simulink model "Subtractor4bit"  (R2025b)
settings: Solver=VariableStepAuto  StartTime=0.0  StopTime=10.0  RelTol=1e-3
settings Model: Creator=cyber  LastModifiedBy=cyber

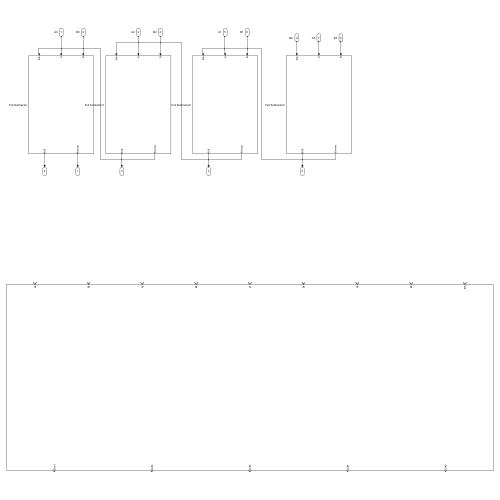
[thumbnail: Simulink's stored preview of the top-level diagram]
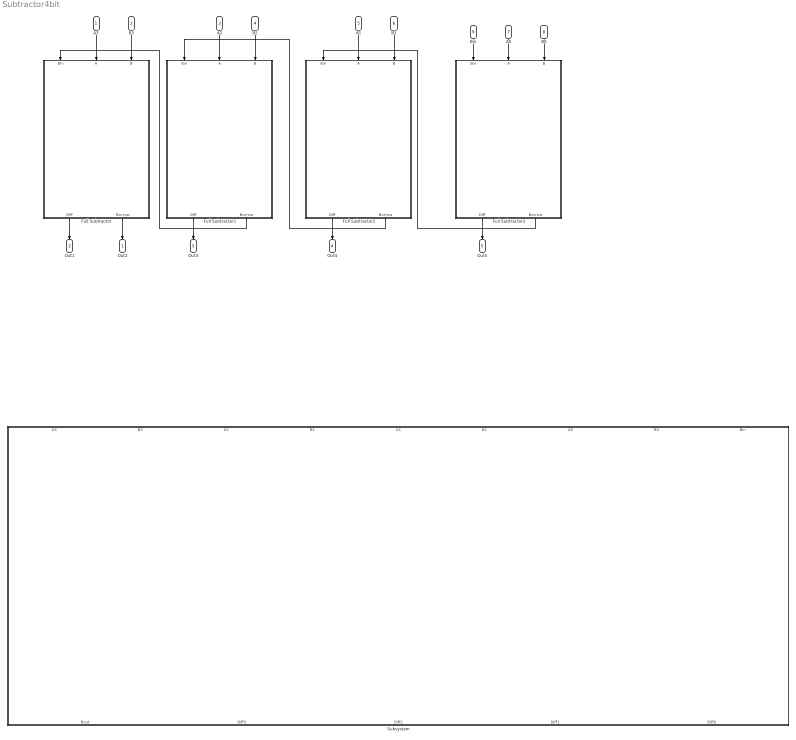
== system Subtractor4bit ==
  A3 : Inport
  B3 : Inport  Port=2
  A2 : Inport  Port=3
  B2 : Inport  Port=4
  A1 : Inport  Port=5
  B1 : Inport  Port=6
  A0 : Inport  Port=7
  B0 : Inport  Port=8
  Bin : Inport  Port=9
  Full Subtractor : Subsystem
  Full Subtractor1 : Subsystem
  Full Subtractor2 : Subsystem
  Full Subtractor3 : Subsystem
  Subsystem : Subsystem
  Out2 : Outport
  Out1 : Outport  Port=2
  Out3 : Outport  Port=3
  Out4 : Outport  Port=4
  Out5 : Outport  Port=5
  wires:
  Full Subtractor/1(Diff) -> Out1/1
  Full Subtractor1/1(Diff) -> Out3/1
  Full Subtractor2/1(Diff) -> Out4/1
  Full Subtractor3/1(Diff) -> Out5/1
  Full Subtractor3/2(Borrow) -> Full Subtractor2/1(Bin)
  Full Subtractor2/2(Borrow) -> Full Subtractor1/1(Bin)
  Full Subtractor1/2(Borrow) -> Full Subtractor/1(Bin)
  A3/1 -> Full Subtractor/2(A)
  B3/1 -> Full Subtractor/3(B)
  A2/1 -> Full Subtractor1/2(A)
  B2/1 -> Full Subtractor1/3(B)
  A1/1 -> Full Subtractor2/2(A)
  B1/1 -> Full Subtractor2/3(B)
  Full Subtractor/2(Borrow) -> Out2/1
  A0/1 -> Full Subtractor3/2(A)
  B0/1 -> Full Subtractor3/3(B)
  Bin/1 -> Full Subtractor3/1(Bin)

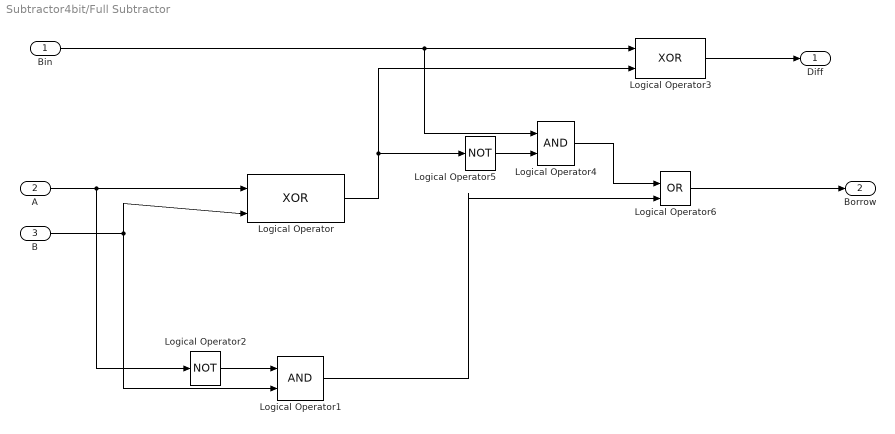
== system Subtractor4bit/Full Subtractor ==
  Bin : Inport
  A : Inport  Port=2
  B : Inport  Port=3
  Logical Operator : Logic  Operator=XOR  IconShape=distinctive  AllPortsSameDT=off  OutDataTypeStr=boolean
  Logical Operator1 : Logic  IconShape=distinctive  AllPortsSameDT=off  OutDataTypeStr=boolean
  Logical Operator2 : Logic  Operator=NOT  IconShape=distinctive  AllPortsSameDT=off  OutDataTypeStr=boolean
  Logical Operator3 : Logic  Operator=XOR  IconShape=distinctive  AllPortsSameDT=off  OutDataTypeStr=boolean
  Logical Operator4 : Logic  IconShape=distinctive  AllPortsSameDT=off  OutDataTypeStr=boolean
  Logical Operator5 : Logic  Operator=NOT  IconShape=distinctive  AllPortsSameDT=off  OutDataTypeStr=boolean
  Logical Operator6 : Logic  Operator=OR  IconShape=distinctive  AllPortsSameDT=off  OutDataTypeStr=boolean
  Diff : Outport
  Borrow : Outport  Port=2
  wires:
  Logical Operator/1 -> Logical Operator3/2, Logical Operator5/1
  Logical Operator1/1 -> Logical Operator6/2
  A/1 -> Logical Operator2/1, Logical Operator/1
  Bin/1 -> Logical Operator4/1, Logical Operator3/1
  Logical Operator3/1 -> Diff/1
  B/1 -> Logical Operator/2, Logical Operator1/2
  Logical Operator2/1 -> Logical Operator1/1
  Logical Operator4/1 -> Logical Operator6/1
  Logical Operator5/1 -> Logical Operator4/2
  Logical Operator6/1 -> Borrow/1

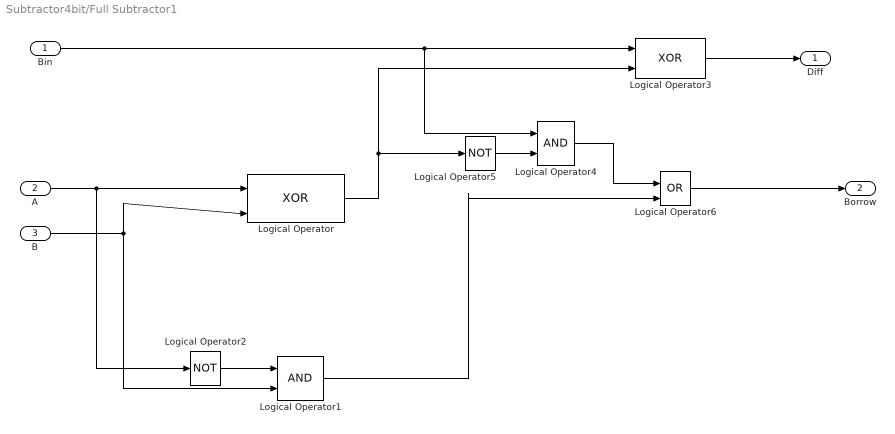
== system Subtractor4bit/Full Subtractor1 ==
  Bin : Inport
  A : Inport  Port=2
  B : Inport  Port=3
  Logical Operator : Logic  Operator=XOR  IconShape=distinctive  AllPortsSameDT=off  OutDataTypeStr=boolean
  Logical Operator1 : Logic  IconShape=distinctive  AllPortsSameDT=off  OutDataTypeStr=boolean
  Logical Operator2 : Logic  Operator=NOT  IconShape=distinctive  AllPortsSameDT=off  OutDataTypeStr=boolean
  Logical Operator3 : Logic  Operator=XOR  IconShape=distinctive  AllPortsSameDT=off  OutDataTypeStr=boolean
  Logical Operator4 : Logic  IconShape=distinctive  AllPortsSameDT=off  OutDataTypeStr=boolean
  Logical Operator5 : Logic  Operator=NOT  IconShape=distinctive  AllPortsSameDT=off  OutDataTypeStr=boolean
  Logical Operator6 : Logic  Operator=OR  IconShape=distinctive  AllPortsSameDT=off  OutDataTypeStr=boolean
  Diff : Outport
  Borrow : Outport  Port=2
  wires:
  Logical Operator/1 -> Logical Operator3/2, Logical Operator5/1
  Logical Operator1/1 -> Logical Operator6/2
  A/1 -> Logical Operator2/1, Logical Operator/1
  Bin/1 -> Logical Operator4/1, Logical Operator3/1
  Logical Operator3/1 -> Diff/1
  B/1 -> Logical Operator/2, Logical Operator1/2
  Logical Operator2/1 -> Logical Operator1/1
  Logical Operator4/1 -> Logical Operator6/1
  Logical Operator5/1 -> Logical Operator4/2
  Logical Operator6/1 -> Borrow/1

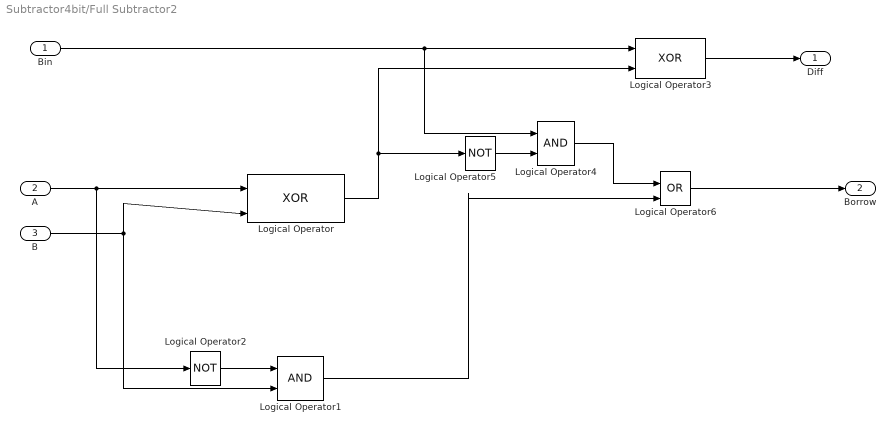
== system Subtractor4bit/Full Subtractor2 ==
  Bin : Inport
  A : Inport  Port=2
  B : Inport  Port=3
  Logical Operator : Logic  Operator=XOR  IconShape=distinctive  AllPortsSameDT=off  OutDataTypeStr=boolean
  Logical Operator1 : Logic  IconShape=distinctive  AllPortsSameDT=off  OutDataTypeStr=boolean
  Logical Operator2 : Logic  Operator=NOT  IconShape=distinctive  AllPortsSameDT=off  OutDataTypeStr=boolean
  Logical Operator3 : Logic  Operator=XOR  IconShape=distinctive  AllPortsSameDT=off  OutDataTypeStr=boolean
  Logical Operator4 : Logic  IconShape=distinctive  AllPortsSameDT=off  OutDataTypeStr=boolean
  Logical Operator5 : Logic  Operator=NOT  IconShape=distinctive  AllPortsSameDT=off  OutDataTypeStr=boolean
  Logical Operator6 : Logic  Operator=OR  IconShape=distinctive  AllPortsSameDT=off  OutDataTypeStr=boolean
  Diff : Outport
  Borrow : Outport  Port=2
  wires:
  Logical Operator/1 -> Logical Operator3/2, Logical Operator5/1
  Logical Operator1/1 -> Logical Operator6/2
  A/1 -> Logical Operator2/1, Logical Operator/1
  Bin/1 -> Logical Operator4/1, Logical Operator3/1
  Logical Operator3/1 -> Diff/1
  B/1 -> Logical Operator/2, Logical Operator1/2
  Logical Operator2/1 -> Logical Operator1/1
  Logical Operator4/1 -> Logical Operator6/1
  Logical Operator5/1 -> Logical Operator4/2
  Logical Operator6/1 -> Borrow/1

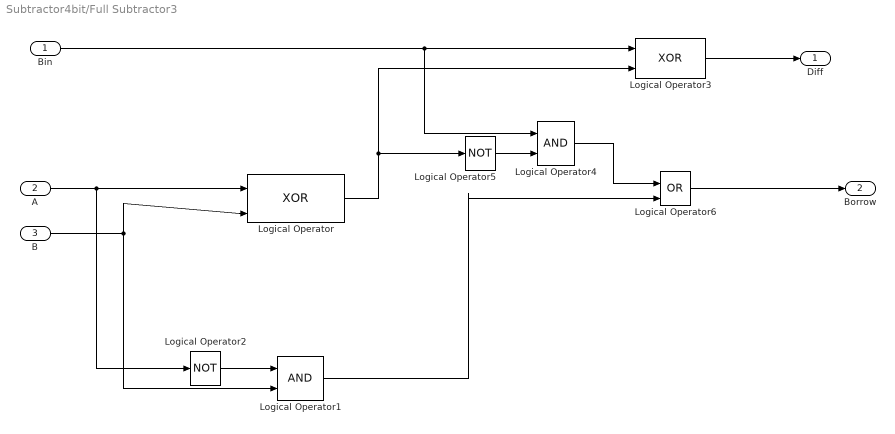
== system Subtractor4bit/Full Subtractor3 ==
  Bin : Inport
  A : Inport  Port=2
  B : Inport  Port=3
  Logical Operator : Logic  Operator=XOR  IconShape=distinctive  AllPortsSameDT=off  OutDataTypeStr=boolean
  Logical Operator1 : Logic  IconShape=distinctive  AllPortsSameDT=off  OutDataTypeStr=boolean
  Logical Operator2 : Logic  Operator=NOT  IconShape=distinctive  AllPortsSameDT=off  OutDataTypeStr=boolean
  Logical Operator3 : Logic  Operator=XOR  IconShape=distinctive  AllPortsSameDT=off  OutDataTypeStr=boolean
  Logical Operator4 : Logic  IconShape=distinctive  AllPortsSameDT=off  OutDataTypeStr=boolean
  Logical Operator5 : Logic  Operator=NOT  IconShape=distinctive  AllPortsSameDT=off  OutDataTypeStr=boolean
  Logical Operator6 : Logic  Operator=OR  IconShape=distinctive  AllPortsSameDT=off  OutDataTypeStr=boolean
  Diff : Outport
  Borrow : Outport  Port=2
  wires:
  Logical Operator/1 -> Logical Operator3/2, Logical Operator5/1
  Logical Operator1/1 -> Logical Operator6/2
  A/1 -> Logical Operator2/1, Logical Operator/1
  Bin/1 -> Logical Operator4/1, Logical Operator3/1
  Logical Operator3/1 -> Diff/1
  B/1 -> Logical Operator/2, Logical Operator1/2
  Logical Operator2/1 -> Logical Operator1/1
  Logical Operator4/1 -> Logical Operator6/1
  Logical Operator5/1 -> Logical Operator4/2
  Logical Operator6/1 -> Borrow/1

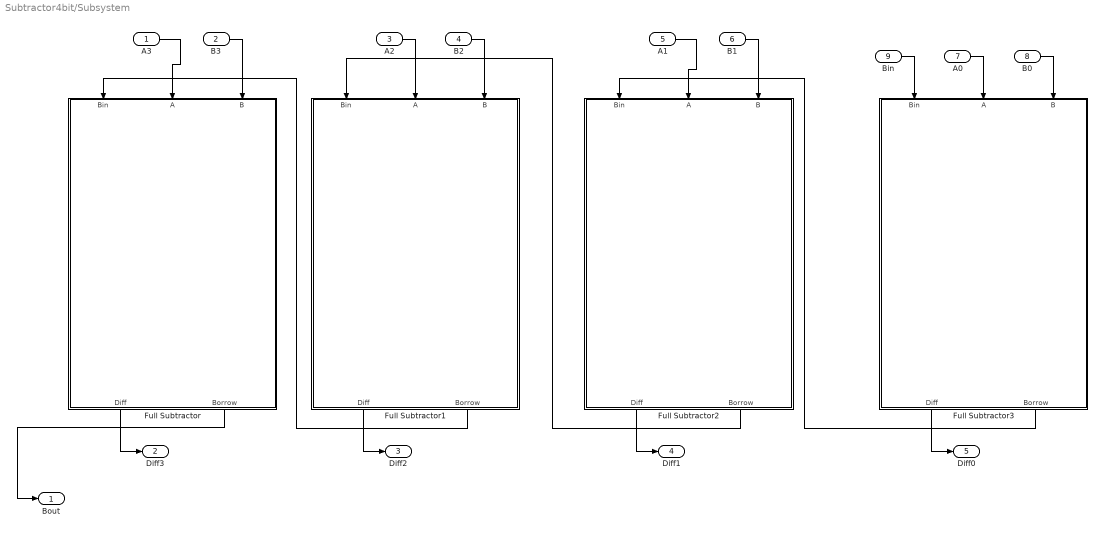
== system Subtractor4bit/Subsystem ==
  A3 : Inport
  B3 : Inport  Port=2
  A2 : Inport  Port=3
  B2 : Inport  Port=4
  A1 : Inport  Port=5
  B1 : Inport  Port=6
  A0 : Inport  Port=7
  B0 : Inport  Port=8
  Bin : Inport  Port=9
  Full Subtractor : Subsystem
  Full Subtractor1 : Subsystem
  Full Subtractor2 : Subsystem
  Full Subtractor3 : Subsystem
  Bout : Outport
  Diff3 : Outport  Port=2
  Diff2 : Outport  Port=3
  Diff1 : Outport  Port=4
  Diff0 : Outport  Port=5
  wires:
  Full Subtractor1/1(Diff) -> Diff2/1
  Full Subtractor2/1(Diff) -> Diff1/1
  Full Subtractor3/2(Borrow) -> Full Subtractor2/1(Bin)
  Full Subtractor2/2(Borrow) -> Full Subtractor1/1(Bin)
  Full Subtractor1/2(Borrow) -> Full Subtractor/1(Bin)
  B3/1 -> Full Subtractor/3(B)
  A0/1 -> Full Subtractor3/2(A)
  A2/1 -> Full Subtractor1/2(A)
  Full Subtractor/2(Borrow) -> Bout/1
  Full Subtractor3/1(Diff) -> Diff0/1
  A3/1 -> Full Subtractor/2(A)
  B2/1 -> Full Subtractor1/3(B)
  A1/1 -> Full Subtractor2/2(A)
  B1/1 -> Full Subtractor2/3(B)
  Bin/1 -> Full Subtractor3/1(Bin)
  Full Subtractor/1(Diff) -> Diff3/1
  B0/1 -> Full Subtractor3/3(B)

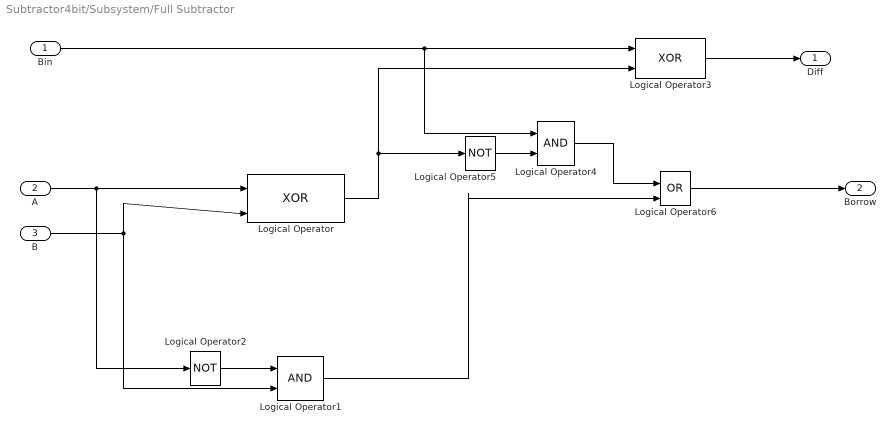
== system Subtractor4bit/Subsystem/Full Subtractor ==
  Bin : Inport
  A : Inport  Port=2
  B : Inport  Port=3
  Logical Operator : Logic  Operator=XOR  IconShape=distinctive  AllPortsSameDT=off  OutDataTypeStr=boolean
  Logical Operator1 : Logic  IconShape=distinctive  AllPortsSameDT=off  OutDataTypeStr=boolean
  Logical Operator2 : Logic  Operator=NOT  IconShape=distinctive  AllPortsSameDT=off  OutDataTypeStr=boolean
  Logical Operator3 : Logic  Operator=XOR  IconShape=distinctive  AllPortsSameDT=off  OutDataTypeStr=boolean
  Logical Operator4 : Logic  IconShape=distinctive  AllPortsSameDT=off  OutDataTypeStr=boolean
  Logical Operator5 : Logic  Operator=NOT  IconShape=distinctive  AllPortsSameDT=off  OutDataTypeStr=boolean
  Logical Operator6 : Logic  Operator=OR  IconShape=distinctive  AllPortsSameDT=off  OutDataTypeStr=boolean
  Diff : Outport
  Borrow : Outport  Port=2
  wires:
  Logical Operator/1 -> Logical Operator3/2, Logical Operator5/1
  Logical Operator1/1 -> Logical Operator6/2
  A/1 -> Logical Operator2/1, Logical Operator/1
  Bin/1 -> Logical Operator4/1, Logical Operator3/1
  Logical Operator3/1 -> Diff/1
  B/1 -> Logical Operator/2, Logical Operator1/2
  Logical Operator2/1 -> Logical Operator1/1
  Logical Operator4/1 -> Logical Operator6/1
  Logical Operator5/1 -> Logical Operator4/2
  Logical Operator6/1 -> Borrow/1

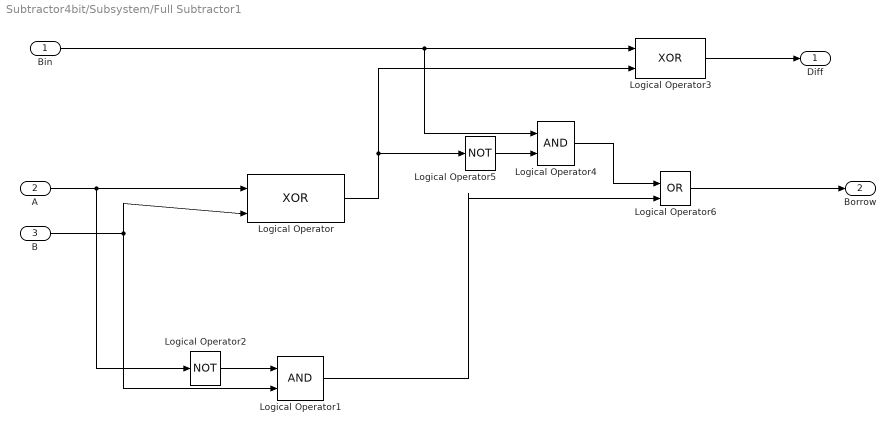
== system Subtractor4bit/Subsystem/Full Subtractor1 ==
  Bin : Inport
  A : Inport  Port=2
  B : Inport  Port=3
  Logical Operator : Logic  Operator=XOR  IconShape=distinctive  AllPortsSameDT=off  OutDataTypeStr=boolean
  Logical Operator1 : Logic  IconShape=distinctive  AllPortsSameDT=off  OutDataTypeStr=boolean
  Logical Operator2 : Logic  Operator=NOT  IconShape=distinctive  AllPortsSameDT=off  OutDataTypeStr=boolean
  Logical Operator3 : Logic  Operator=XOR  IconShape=distinctive  AllPortsSameDT=off  OutDataTypeStr=boolean
  Logical Operator4 : Logic  IconShape=distinctive  AllPortsSameDT=off  OutDataTypeStr=boolean
  Logical Operator5 : Logic  Operator=NOT  IconShape=distinctive  AllPortsSameDT=off  OutDataTypeStr=boolean
  Logical Operator6 : Logic  Operator=OR  IconShape=distinctive  AllPortsSameDT=off  OutDataTypeStr=boolean
  Diff : Outport
  Borrow : Outport  Port=2
  wires:
  Logical Operator/1 -> Logical Operator3/2, Logical Operator5/1
  Logical Operator1/1 -> Logical Operator6/2
  A/1 -> Logical Operator2/1, Logical Operator/1
  Bin/1 -> Logical Operator4/1, Logical Operator3/1
  Logical Operator3/1 -> Diff/1
  B/1 -> Logical Operator/2, Logical Operator1/2
  Logical Operator2/1 -> Logical Operator1/1
  Logical Operator4/1 -> Logical Operator6/1
  Logical Operator5/1 -> Logical Operator4/2
  Logical Operator6/1 -> Borrow/1

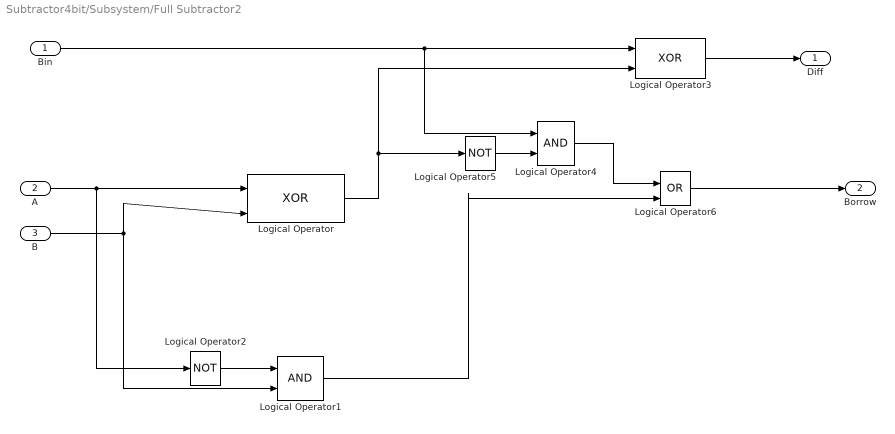
== system Subtractor4bit/Subsystem/Full Subtractor2 ==
  Bin : Inport
  A : Inport  Port=2
  B : Inport  Port=3
  Logical Operator : Logic  Operator=XOR  IconShape=distinctive  AllPortsSameDT=off  OutDataTypeStr=boolean
  Logical Operator1 : Logic  IconShape=distinctive  AllPortsSameDT=off  OutDataTypeStr=boolean
  Logical Operator2 : Logic  Operator=NOT  IconShape=distinctive  AllPortsSameDT=off  OutDataTypeStr=boolean
  Logical Operator3 : Logic  Operator=XOR  IconShape=distinctive  AllPortsSameDT=off  OutDataTypeStr=boolean
  Logical Operator4 : Logic  IconShape=distinctive  AllPortsSameDT=off  OutDataTypeStr=boolean
  Logical Operator5 : Logic  Operator=NOT  IconShape=distinctive  AllPortsSameDT=off  OutDataTypeStr=boolean
  Logical Operator6 : Logic  Operator=OR  IconShape=distinctive  AllPortsSameDT=off  OutDataTypeStr=boolean
  Diff : Outport
  Borrow : Outport  Port=2
  wires:
  Logical Operator/1 -> Logical Operator3/2, Logical Operator5/1
  Logical Operator1/1 -> Logical Operator6/2
  A/1 -> Logical Operator2/1, Logical Operator/1
  Bin/1 -> Logical Operator4/1, Logical Operator3/1
  Logical Operator3/1 -> Diff/1
  B/1 -> Logical Operator/2, Logical Operator1/2
  Logical Operator2/1 -> Logical Operator1/1
  Logical Operator4/1 -> Logical Operator6/1
  Logical Operator5/1 -> Logical Operator4/2
  Logical Operator6/1 -> Borrow/1

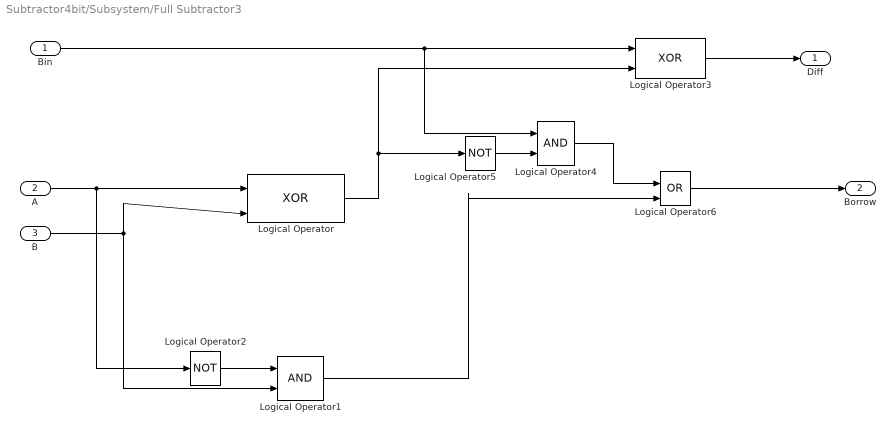
== system Subtractor4bit/Subsystem/Full Subtractor3 ==
  Bin : Inport
  A : Inport  Port=2
  B : Inport  Port=3
  Logical Operator : Logic  Operator=XOR  IconShape=distinctive  AllPortsSameDT=off  OutDataTypeStr=boolean
  Logical Operator1 : Logic  IconShape=distinctive  AllPortsSameDT=off  OutDataTypeStr=boolean
  Logical Operator2 : Logic  Operator=NOT  IconShape=distinctive  AllPortsSameDT=off  OutDataTypeStr=boolean
  Logical Operator3 : Logic  Operator=XOR  IconShape=distinctive  AllPortsSameDT=off  OutDataTypeStr=boolean
  Logical Operator4 : Logic  IconShape=distinctive  AllPortsSameDT=off  OutDataTypeStr=boolean
  Logical Operator5 : Logic  Operator=NOT  IconShape=distinctive  AllPortsSameDT=off  OutDataTypeStr=boolean
  Logical Operator6 : Logic  Operator=OR  IconShape=distinctive  AllPortsSameDT=off  OutDataTypeStr=boolean
  Diff : Outport
  Borrow : Outport  Port=2
  wires:
  Logical Operator/1 -> Logical Operator3/2, Logical Operator5/1
  Logical Operator1/1 -> Logical Operator6/2
  A/1 -> Logical Operator2/1, Logical Operator/1
  Bin/1 -> Logical Operator4/1, Logical Operator3/1
  Logical Operator3/1 -> Diff/1
  B/1 -> Logical Operator/2, Logical Operator1/2
  Logical Operator2/1 -> Logical Operator1/1
  Logical Operator4/1 -> Logical Operator6/1
  Logical Operator5/1 -> Logical Operator4/2
  Logical Operator6/1 -> Borrow/1
